simulink model "Lag_Pole_Cancellation"  (R2022b)
settings: Solver=VariableStepAuto  StartTime=0.0  StopTime=15  RelTol=1e-3
libraries: simulink x3
settings Model: Creator=amirz  LastModifiedBy=amirz

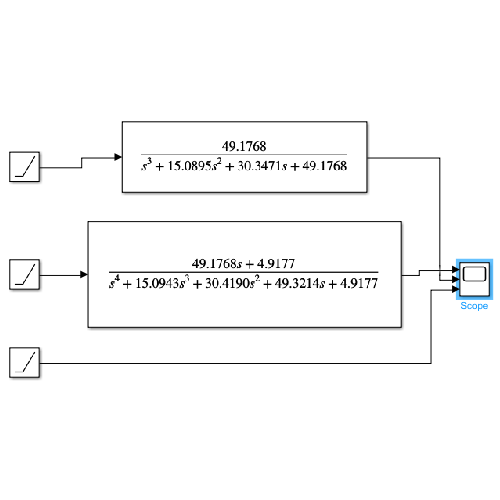
[thumbnail: Simulink's stored preview of the top-level diagram]
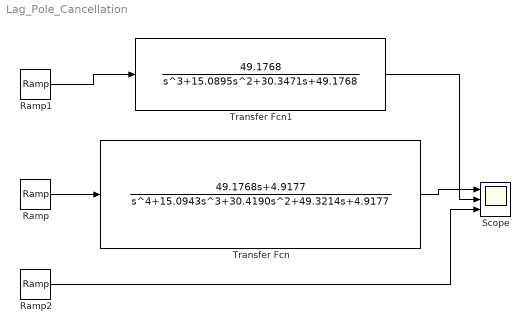
== system Lag_Pole_Cancellation ==
  Ramp : simulink/Sources/Ramp  slope=1  start=0  InitialOutput=0
  Ramp1 : simulink/Sources/Ramp  slope=1  start=0  InitialOutput=0
  Ramp2 : simulink/Sources/Ramp  slope=1  start=0  InitialOutput=0
  Scope : Scope  NumInputPorts=3
  Transfer Fcn : TransferFcn  Numerator=[49.1768 4.9177]  Denominator=[1 15.0943 30.4190 49.3214 4.9177]
  Transfer Fcn1 : TransferFcn  Numerator=[49.1768]  Denominator=[1 15.0895 30.3471 49.1768]
  wires:
  Ramp/1 -> Transfer Fcn/1
  Transfer Fcn/1 -> Scope/1
  Transfer Fcn1/1 -> Scope/2
  Ramp1/1 -> Transfer Fcn1/1
  Ramp2/1 -> Scope/3
